simulink library "Lateral_Controllers"  (R2021a)
settings: Solver=VariableStepAuto  StartTime=0.0  StopTime=10.0  RelTol=1e-3
undefined symbols (not defined in the file or in its folder): Vehicle_id, Vehicles
libraries: robotalgslib x1, drivingvehiclecontroller x1
settings Model: Creator=Laura Slabon  LastModifiedBy=Laura Slabon

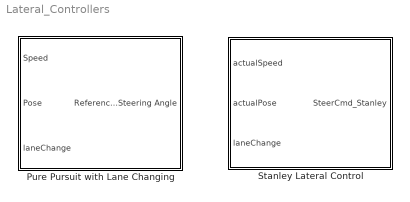
== system Lateral_Controllers ==
  Pure Pursuit with Lane Changing : Subsystem
  Stanley Lateral Control : Subsystem

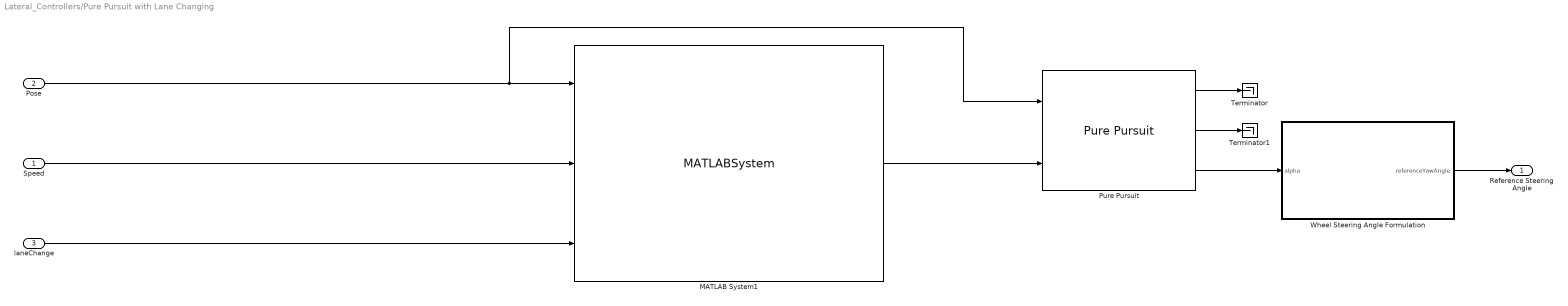
== system Lateral_Controllers/Pure Pursuit with Lane Changing ==
  Speed : Inport
  Pose : Inport  Port=2
  laneChange : Inport  Port=3
  MATLAB System1 : MATLABSystem  System=PurePursuit_WPGenerator  Vehicle_id=Vehicle_id  SimulateUsing=Interpreted execution
      mask Type: PurePursuit_WPGenerator
      mask Display:
      | image('WaypointGenerator.png');
      | port_label('input',1,'pose');
      | port_label('input',2,'speed');
      | port_label('input',3,'changeLane');
      | port_label('output',1,'nextWPs');
  Pure Pursuit : robotalgslib/Pure Pursuit  DesiredLinearVelocity=Vehicles(Vehicle_id).dynamics.maxSpeed  MaxAngularVelocity=1  LookaheadDistance=6  TargetDirPort=on  SimulateUsing=Code generation
  Terminator : Terminator
  Terminator1 : Terminator
  Wheel Steering Angle Formulation : Subsystem
  Reference Steering Angle : Outport
  wires:
  laneChange/1 -> MATLAB System1/3
  Speed/1 -> MATLAB System1/2
  Pose/1 -> Pure Pursuit/1, MATLAB System1/1
  Pure Pursuit/1 -> Terminator/1
  Pure Pursuit/2 -> Terminator1/1
  Pure Pursuit/3 -> Wheel Steering Angle Formulation/1(alpha)
  Wheel Steering Angle Formulation/1(referenceYawAngle) -> Reference Steering Angle/1
  MATLAB System1/1 -> Pure Pursuit/2

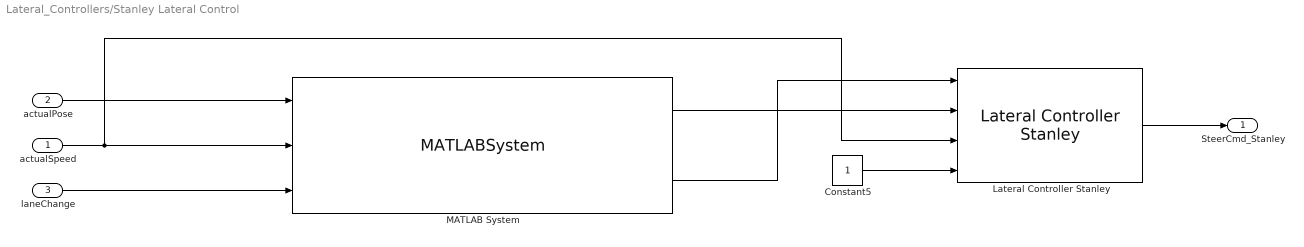
== system Lateral_Controllers/Stanley Lateral Control ==
  actualSpeed : Inport
  actualPose : Inport  Port=2
  laneChange : Inport  Port=3
  Constant5 : Constant
  Lateral Controller Stanley : drivingvehiclecontroller/Lateral Controller Stanley  ModelType=Kinematic bicycle model  PositionGainF=2.5  PositionGainR=2.5  YawRateGain=0.2  DelayGain=0.2  VehicleMass=1575  Lf=1.2  Lr=1.6  TireStiffness=19000  Wheelbase=3  MaxSteeringAngle=35
      settings: SourceProductBaseCode=DR
  MATLAB System : MATLABSystem  System=V_WPGenerator_Stanley  Vehicle_id=Vehicle_id  SimulateUsing=Interpreted execution
      mask Type: V_WPGenerator_Stanley
      mask Display:
      | image('WaypointGenerator.png');
      | port_label('input',1,'pose');
      | port_label('input',2,'speed');
      | port_label('input',3,'changeLane');
      | port_label('output',1,'poseOut');
      | port_label('output',2,'referencePose');
  SteerCmd_Stanley : Outport
  wires:
  actualPose/1 -> MATLAB System/1
  MATLAB System/1 -> Lateral Controller Stanley/2
  actualSpeed/1 -> Lateral Controller Stanley/3, MATLAB System/2
  Constant5/1 -> Lateral Controller Stanley/4
  MATLAB System/2 -> Lateral Controller Stanley/1
  Lateral Controller Stanley/1 -> SteerCmd_Stanley/1
  laneChange/1 -> MATLAB System/3

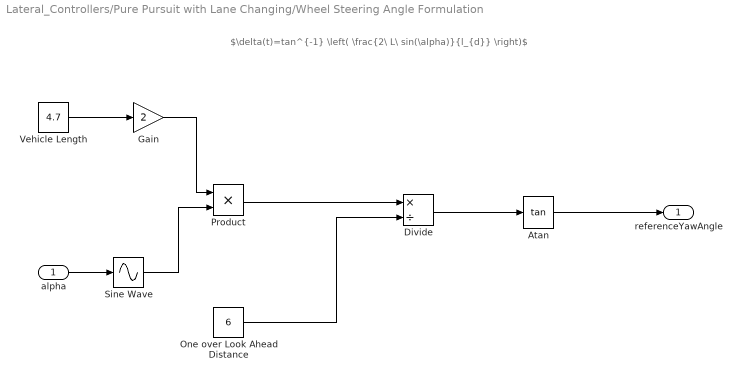
== system Lateral_Controllers/Pure Pursuit with Lane Changing/Wheel Steering Angle Formulation ==
  note: $\delta(t)=tan^{-1} \left( \frac{2\ L\ sin(\alpha)}{l_{d}} \right)$
  alpha : Inport
  Atan : Trigonometry  Operator=tan
  Divide : Product  Inputs=*/
  Gain : Gain  Gain=2
  One over Look Ahead Distance : Constant  Value=6
  Product : Product
  Sine Wave : Sin  TimeSource=Use external signal  SampleTime=0
  Vehicle Length : Constant  Value=4.7
  referenceYawAngle : Outport
  wires:
  Vehicle Length/1 -> Gain/1
  Gain/1 -> Product/1
  alpha/1 -> Sine Wave/1
  Sine Wave/1 -> Product/2
  Product/1 -> Divide/1
  One over Look Ahead Distance/1 -> Divide/2
  Divide/1 -> Atan/1
  Atan/1 -> referenceYawAngle/1
